simulink model "meanfit"  (R2018a)
settings: Solver=FixedStepDiscrete  StartTime=t(1)  StopTime=t(end)  RelTol=1e-3  EnableMultiTasking=on
PreLoadFcn:
  | data = xlsread('temp.xls');
  | t = data(:,1);
  | u = data(:,2);
settings Model: Creator=jrivitus  LastModifiedBy=bneiswan
settings DataIOCC: LimitDataPoints=on  LoadExternalInput=on  SaveFormat=Array
settings OptimizationCC: ExpressionDepthLimit=2147483647  InitFltsAndDblsToZero=on  LifeSpan=inf
settings DebuggingCC: UnderspecifiedInitializationDetection=Classic  MergeDetectMultiDrivingBlocksExec=none  ParameterPrecisionLossMsg=none  FcnCallInpInsideContextMsg=warning  AllowSymbolicDim=off  StateNameClashWarn=warning  SFUnexpectedBacktrackingDiag=warning  SFNoUnconditionalDefaultTransitionDiag=warning  SFExecutionAtInitializationDiag=none
settings HardwareCC: ProdBitPerPointer=32  ProdBitPerSizeT=32  ProdBitPerPtrDiffT=32  ProdLargestAtomicFloat=None  ProdIntDivRoundTo=Undefined  ProdEndianess=Unspecified  ProdWordSize=32  ProdHWDeviceType=32-bit Generic
settings ModelReferenceCC: PropagateSignalLabelsOutOfModel=off
settings CodeAppCC: StateflowObjectComments=on
settings GRTTargetCC: TargetLangStandard=C89/C90 (ANSI)  GeneratePreprocessorConditionals=Disable all  CombineOutputUpdateFcns=off  GRTInterface=on
settings ConfigComp: CovMetricSettings=dw  CovHtmlReporting=on  CovSaveCumulativeToWorkspaceVar=on  CovSaveSingleToWorkspaceVar=on  CovExternalEMLEnable=off  CovSFcnEnable=off

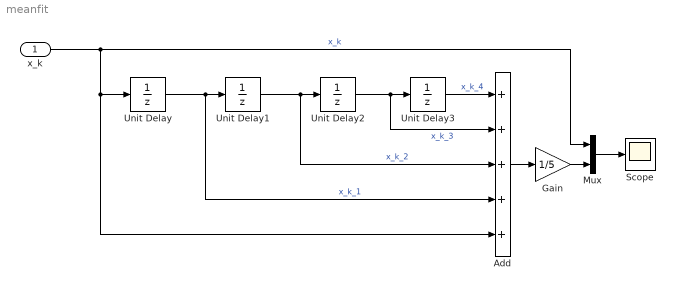
== system meanfit ==
  x_k : Inport
  Add : Sum  Inputs=+++++
  Gain : Gain  Gain=1/5
  Mux : Mux  Inputs=2
  Scope : Scope
  Unit Delay{,1..3} (4 alike) : UnitDelay
  wires:
  x_k/1 -> Mux/1, Add/5, Unit Delay/1  "x_k"
  Unit Delay/1 -> Unit Delay1/1, Add/4  "x_k_1"
  Unit Delay1/1 -> Unit Delay2/1, Add/3  "x_k_2"
  Unit Delay2/1 -> Unit Delay3/1, Add/2  "x_k_3"
  Unit Delay3/1 -> Add/1  "x_k_4"
  Add/1 -> Gain/1
  Gain/1 -> Mux/2
  Mux/1 -> Scope/1
